simulink model "simldisk"  (R2017b)
settings: Solver=FixedStepDiscrete  StartTime=0.0  StopTime=10.0  FixedStep=Ts  RelTol=1e-3  EnableMultiTasking=on
values from neighbouring files (symbols this model uses):
  A = [1 0 0 0 0.01 1 0 0 -9.79521061044e-05 -0.0195804527741 1.00293856318 0.587413583222 ... (16 elements, 4x4)]    [diskretnySM2.mat]    (also in simdiskkyvadlo.m = expm(Ac*Ts); sysd.mat = [1 0 0 0 0.01 1 0 0 -9.7856100623e-05 -0.0195420736082 0.997; sysd2.mat)
  B = [0.00012496859202 0.0249916014216 -0.000624057760604 -0.124748042648]    [diskretnySM2.mat]    (also in simdiskkyvadlo.m = Ac\(A-eye(length(A)))*Bc; sysd.mat = [0.000124948203496 0.0249834509022 0.000623446104887 0.12450; sysd2.mat)
  C = [1  0  0  0; 0  0  1  0]    [diskretnySM2.mat]    (also in sysd.mat; sysd2.mat)
  D = [0 0]    [diskretnySM2.mat]    (also in sysd.mat; sysd2.mat)
  dx0 = x0-xlin    [kalmankyvadlo.m]    (also in simEKFkyvadlo.m; simKFkyvadlo.m = zeros(nx,1); simdiskkyvadlo.m = [0;0;0;0]; simlinkyvadlo.m = [0;0;-pi/6;0])
libraries: simulink_need_slupdate x1
settings Model: Creator=gulan  LastModifiedBy=gulan
settings OptimizationCC: LifeSpan=inf
settings DebuggingCC: SFUnexpectedBacktrackingDiag=warning  SFNoUnconditionalDefaultTransitionDiag=warning  SFExecutionAtInitializationDiag=none
settings CodeAppCC: StateflowObjectComments=on
settings GRTTargetCC: TargetLangStandard=C89/C90 (ANSI)  GeneratePreprocessorConditionals=Disable all
settings ConfigComp: CovMetricSettings=dw  CovHtmlReporting=on  CovSaveCumulativeToWorkspaceVar=on  CovSaveSingleToWorkspaceVar=on  CovExternalEMLEnable=off

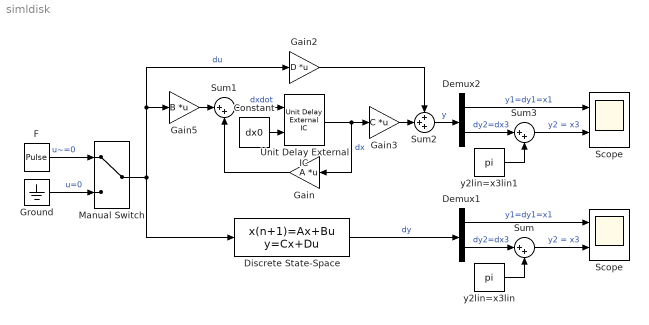
== system simldisk ==
  " Scope" : Scope  NumInputPorts=2
  " Scope " : Scope  NumInputPorts=2
  Constant : Constant  Value=dx0  SampleTime=0.01
  Demux1 : Demux  Outputs=2
  Demux2 : Demux  Outputs=2
  Discrete State-Space : DiscreteStateSpace  A=A  B=B  C=C  D=D  InitialCondition=dx0  SampleTime=-1
  F : DiscretePulseGenerator  PulseType=Time based  Amplitude=50  Period=10  PulseWidth=0.1
  Gain : Gain  Gain=A  Multiplication=Matrix(K*u) (u vector)
  Gain2 : Gain  Gain=D  Multiplication=Matrix(K*u) (u vector)
  Gain3 : Gain  Gain=C  Multiplication=Matrix(K*u) (u vector)
  "Gain5 " : Gain  Gain=B  Multiplication=Matrix(K*u) (u vector)
  Ground : Ground
  Manual Switch : ManualSwitch
  Sum : Sum  Inputs=|++
  Sum1 : Sum  Inputs=|++
  Sum2 : Sum  Inputs=+++
  Sum3 : Sum  Inputs=|++
  Unit Delay External IC : simulink_need_slupdate/Unit Delay External IC  tsamp=-1
      settings: SourceProductName=Simulink  SourceProductBaseCode=SL
  y2lin=x3lin : Constant  Value=pi
  y2lin=x3lin1 : Constant  Value=pi
  wires:
  F/1 -> Manual Switch/1  "u~=0"
  Manual Switch/1 -> Discrete State-Space/1, Gain2/1, "Gain5 "/1  "du"
  Demux1/1 -> " Scope"/1  "y1=dy1=x1"
  Demux1/2 -> Sum/1  "dy2=dx3"
  Sum/1 -> " Scope"/2  "y2 = x3"
  y2lin=x3lin/1 -> Sum/2
  Gain/1 -> Sum1/2
  "Gain5 "/1 -> Sum1/1
  Sum1/1 -> Unit Delay External IC/1  "dxdot"
  Constant/1 -> Unit Delay External IC/2
  Unit Delay External IC/1 -> Gain3/1, Gain/1  "dx"
  Gain2/1 -> Sum2/1
  Gain3/1 -> Sum2/2
  Demux2/1 -> " Scope "/1  "y1=dy1=x1"
  Demux2/2 -> Sum3/1  "dy2=dx3"
  Sum3/1 -> " Scope "/2  "y2 = x3"
  y2lin=x3lin1/1 -> Sum3/2
  Sum2/1 -> Demux2/1  "y"
  Ground/1 -> Manual Switch/2  "u=0"
  Discrete State-Space/1 -> Demux1/1  "dy"
